simulink library "SampleRateConverterBtc"  (R2022b)
settings: Solver=VariableStepAuto  StartTime=0.0  StopTime=10.0  RelTol=1e-3
undefined symbols (not defined in the file or in its folder): __PRM__SERIALIZED__DATA__, ADVANCE_VEC, COEFFICIENTS, SRC
libraries: HandyTextFile x2
settings Model: Creator=kl13806  LastModifiedBy=kl13806
settings SolverCC: AlgebraicLoopSolver=TrustRegion
settings DebuggingCC: UnconnectedInputMsg=warning  UnconnectedOutputMsg=warning  UnconnectedLineMsg=warning  SFMachineParentedDataDiag=warning
settings ModelReferenceCC: EnableRefExpFcnMdlSchedulingChecks=on
settings RTWCC: DLArmComputeVersion=19.05

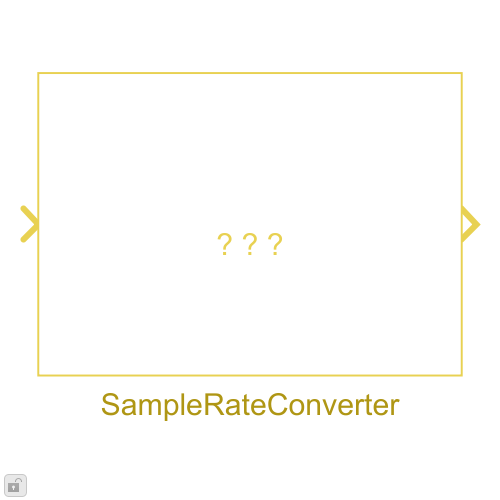
[thumbnail: Simulink's stored preview of the top-level diagram]
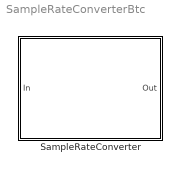
== system SampleRateConverterBtc ==
  SampleRateConverter : Subsystem  BlockKeywords=__PRM__SERIALIZED__DATA__:SRC  mask(Blocklib SampleRateConverter){Config=[]}
      mask prompts: Config "SampleRateConverterConfig"
      mask help: This block resamples the input frame signal for a specified fractional rate.
      mask init:
      | blkh=gcbh;
      | Config=BTConfig.Assert(blkh,Config);
      | Config.Validate();
      | 
      | [COEFFICIENTS, ADVANCE_VEC, BLOCKSIZE] = SampleRateConverter_init(...
      |    Config.Upfactor, Config.Downfactor, Config.RateSelector, ...
      |        Config.Fs, Config.FPassband, Config.FHearing, ...
      |        Config.PassbandRipple, Config.StopbandAttenuation);
      mask Display: fprintf('%d/%d SRC', Config.Upfactor, Config.Downfactor)

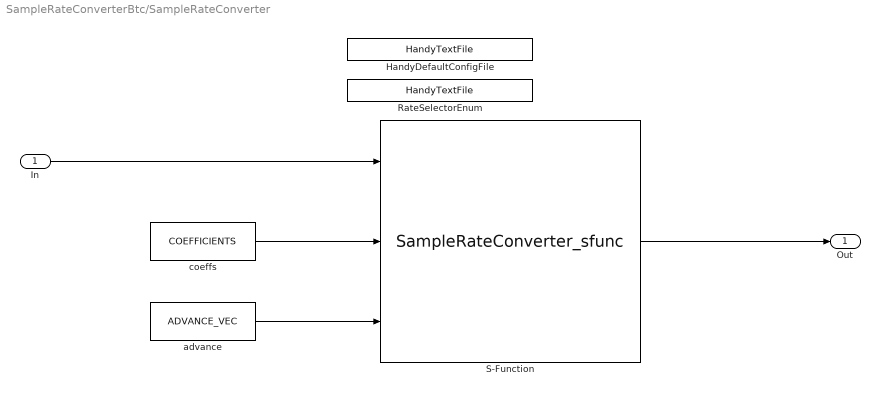
== system SampleRateConverterBtc/SampleRateConverter ==
  In : Inport
  HandyDefaultConfigFile : HandyTextFile/HandyTextFile  TemplateSource=Config  FileSuffix=Init  OpenDialogOnLoad=off  UseThisBlockName=off  TheDefaultText=|  ShowInLibBrowser=on
      | % $(FILENAME) Setup model parameters for each "Init" callback (e.g. update diagram)
      | sample_rate_in_hertz = 44100;
      | frame_size = 32;
      | sysin_channel_count = 2;
  RateSelectorEnum : HandyTextFile/HandyTextFile  TemplateSource=Enum  FileSuffix=Init  OpenDialogOnLoad=off  UseThisBlockName=on  TheDefaultText=|  ShowInLibBrowser=on
      | % $(FILENAME) Setup model parameters for each "Init" callback (e.g. update diagram)
      | sample_rate_in_hertz = 44100;
      | frame_size = 32;
      | sysin_channel_count = 2;
  S-Function : S-Function  FunctionName=SampleRateConverter_sfunc  Parameters=Config.Upfactor, Config.Downfactor, Config.OutFrameSize, BLOCKSIZE  SFunctionDeploymentMode=off  EnableBusSupport=off
  advance : Constant  Value=ADVANCE_VEC  VectorParams1D=off  OutDataTypeStr=int32  SampleTime=-1
  coeffs : Constant  Value=COEFFICIENTS  VectorParams1D=off  OutDataTypeStr=single  SampleTime=-1
  Out : Outport  VectorParamsAs1DForOutWhenUnconnected=off
  wires:
  advance/1 -> S-Function/3
  coeffs/1 -> S-Function/2
  S-Function/1 -> Out/1
  In/1 -> S-Function/1
